simulink model "F16_dynamic_model_2019a"  (R2024b)
settings: Solver=ode3  StartTime=0.0  StopTime=1  FixedStep=1/1000  RelTol=1e-3
values from neighbouring files (symbols this model uses):
  f16data =     [f16aerodata.mat]
  f16engine =     [f16engine.mat]
undefined symbols (not defined in the file or in its folder): e0_0, e1_0, e2_0, e3_0, Earth, ft, m, s, WGS84
libraries: simulink_extras x11, simulink x7, aerosimlib x5, vrlib x3, sharedtransform x3, aerolibfltsims x3, slpidlib x3, aerolibconvert2 x2, aerolibutil x1, sharedutil x1, shared6dof x1, aerolibtransform2 x1
(part 2 of 3)

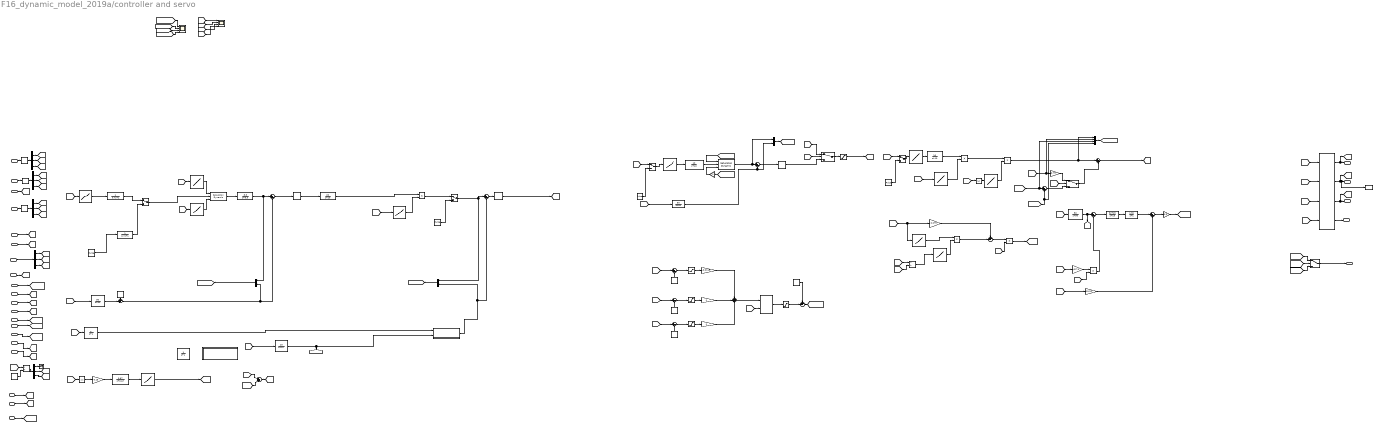
== system F16_dynamic_model_2019a/controller and servo  ==
  note: G limiters CAT 1
  note: Gain Scheduled Pitch Rate
  note: Scope
  note: Pitch Rate feedback
  note: Normal Acceleration feedback
  note: Adverse Yaw Prevent
  note: Stability Augmentation System
  note: INPUTS
  note: - PITCH CONTROL -
  note: POWER CONTROL
  note: SERVO (SIMPLE ACTUATORS)
  note: - RUDDER CONTROL -
  note: - ROLL CONTROL -
  note: Fake Alpha For High Roll to Alpha Limiter
  note: Roll Departure Preventation
  note: Aileron Rudder Interconnect ( ARI)
  note: NOT: Hız (160-255m/s arası) arttıkça
      |  command gain azalıyor.
  wbdots : Inport
  phithetapsi : Inport  Port=2
  h : Inport  Port=3
  wb (rad/s) : Inport  Port=4
  "Beta " : Inport  Port=5
  Vr : Inport  Port=6
  Ve : Inport  Port=7
  AoA : Inport  Port=8
  q_ah_des : Inport  Port=9
  dpower_ah : Inport  Port=10
  de_j : Inport  Port=11
  da_j : Inport  Port=12
  dr_j : Inport  Port=13
  dpower_j : Inport  Port=14
  "ah_check " : Inport  Port=15
  speedb : Inport  Port=16
  Ab(m/s2) : Inport  Port=17
  q_dyn : Inport  Port=18
  p_static : Inport  Port=19
  "turn_check " : Inport  Port=20
  1-D Lookup Table : Lookup_n-D  NumberOfTableDimensions=1  BreakpointsForDimension1=[-1, -0.2, 0.2, 1]  Table=[-30, 0, 0, 30]  ExtrapMethod=Clip  UseLastTableValue=on  InternalRulePriority=Speed  RndMeth=Simplest
  1-D Lookup Table1 : Lookup_n-D  NumberOfTableDimensions=1  BreakpointsForDimension1=[20, 30]  Table=[1, 0]  ExtrapMethod=Clip  UseLastTableValue=on  InternalRulePriority=Speed  RndMeth=Simplest
  1-D Lookup Table2 : Lookup_n-D  NumberOfTableDimensions=1  BreakpointsForDimension1=[3, 8.4]  Table=[0, 5.4]  ExtrapMethod=Clip  UseLastTableValue=on  InternalRulePriority=Speed  RndMeth=Simplest
  1-D Lookup Table3 : Lookup_n-D  NumberOfTableDimensions=1  BreakpointsForDimension1=[-10, 0, 10]  Table=[0, 1, 0]  ExtrapMethod=Clip  UseLastTableValue=on  InternalRulePriority=Speed  RndMeth=Simplest
  1-D Lookup Table4 : Lookup_n-D  NumberOfTableDimensions=1  BreakpointsForDimension1=[0.187, 1.129]  Table=[0, 1]  ExtrapMethod=Clip  UseLastTableValue=on  InternalRulePriority=Speed  RndMeth=Simplest
  Abs : Abs  SaturateOnIntegerOverflow=off
  Abs1 : Abs  SaturateOnIntegerOverflow=off
  Constant : Constant  Value=9.81
  Constant2 : Constant  Value=10500
  Constant3 : Constant  Value=15
  Constant4 : Constant  Value=5
  Constant5 : Constant  Value=308
  Control Signals : Scope  NumInputPorts=4
  Demux{,1..4} (5 alike) : Demux  Outputs=3
  Gain Scheduling Pitch Rate Feedback : Subsystem
  Gain1 : Gain  Gain=0.15
  Gain2 : Gain  Gain=-1
  Gain3 : Gain  Gain=0.75
  Manual Switch{,1..3} (4 alike) : ManualSwitch
  Multiply : Gain  Gain=-0.0115
  Multiply2 : Gain  Gain=0.075
  Multiply3 : Gain  Gain=4
  Multiply4 : Gain  Gain=4
  Multiply5 : Gain  Gain=1/57.3
  Multiply6 : Gain  Gain=19.32
  Multiply7 : Gain  Gain=0.5
  Mux : Mux  Inputs=2
  Mux1 : Mux  Inputs=2
  Mux2 : Mux  Inputs=2
  Mux3 : Mux
  PID Controller1 : slpidlib/PID Controller  Controller=PID  Form=Parallel  TimeDomain=Continuous-time  UseExternalTs=off  SampleTime=-1  IntegratorMethod=Forward Euler  FilterMethod=Forward Euler  ControllerParametersSource=internal  P=0.35  I=0.8  UseKiTs=off  D=0.04  UseExternalDerivativeSource=off  N=100  UseFilter=on  TunerSelectOption=Transfer Function Based (PID Tuner App)  InitialConditionSource=internal  InitialConditionForIntegrator=0  InitialConditionForFilter=0  DifferentiatorICPrevScaledInput=0  ExternalReset=none  TrackingMode=off  Kt=1  LimitOutput=on  SatLimitsSource=internal  UpperSaturationLimit=21.5  LowerSaturationLimit=-21.5  LinearizeAsGain=on  AntiWindupMode=clamping  Kb=1  LimitIntegrator=off  UpperIntegratorSaturationLimit=inf  LowerIntegratorSaturationLimit=-inf  POutMin=[]  POutMax=[]  IOutMin=[]  IOutMax=[]  DOutMin=[]  DOutMax=[]  NOutMin=[]  NOutMax=[]  SumOutMin=[]  SumOutMax=[]  SaturationOutMin=[]  SaturationOutMax=[]  PParamMin=[]  PParamMax=[]  IParamMin=[]  IParamMax=[]  DParamMin=[]  DParamMax=[]  NParamMin=[]  NParamMax=[]  KbParamMin=[]  KbParamMax=[]  KtParamMin=[]  KtParamMax=[]  KbOutMin=[]  KbOutMax=[]  KtOutMin=[]  KtOutMax=[]  IntegratorOutMin=[]  IntegratorOutMax=[]  FilterOutMin=[]  FilterOutMax=[]  SumI1OutMin=[]  SumI1OutMax=[]  SumI2OutMin=[]  SumI2OutMax=[]  SumI3OutMin=[]  SumI3OutMax=[]  SumI4OutMin=[]  SumI4OutMax=[]  SumDOutMin=[]  SumDOutMax=[]  DifferentiatorOutMin=[]  DifferentiatorOutMax=[]  FilterDiffOutCoefMin=[]  FilterDiffOutCoefMax=[]  ReciprocalOutMin=[]  ReciprocalOutMax=[]  SumDenOutMin=[]  SumDenOutMax=[]  SumNumOutMin=[]  SumNumOutMax=[]  DivideOutMin=[]  DivideOutMax=[]  UdiffTsProdOutMin=[]  UdiffTsProdOutMax=[]  NTsProdOutMin=[]  NTsProdOutMax=[]  UintegralTsProdOutMin=[]  UintegralTsProdOutMax=[]  UngainTsProdOutMin=[]  UngainTsProdOutMax=[]  ClampingZeroOutDataTypeStr=Inherit: Inherit via back propagation  ClampingZeroOutMin=[]  ClampingZeroOutMax=[]  FilterDenConstantOutDataTypeStr=Inherit: Inherit via back propagation  FilterDenConstantOutMin=[]  FilterDenConstantOutMax=[]  PCopyOutDataTypeStr=Inherit: Inherit via back propagation  PCopyOutMin=[]  PCopyOutMax=[]  NCopyOutDataTypeStr=Inherit: Inherit via back propagation  NCopyOutMin=[]  NCopyOutMax=[]  IntegratorContinuousStateAttributes=''  IntegratorStateMustResolveToSignalObject=off  IntegratorRTWStateStorageClass=Auto  FilterContinuousStateAttributes=''  FilterStateMustResolveToSignalObject=off  FilterRTWStateStorageClass=Auto  ParallelPVariant=InternalParameters  IdealPVariant=Disabled  IVariant=InternalParameters  DVariant=InternalParameters  IntegratorVariant=Continuous  SatVariant=Enabled  AWVariant=ContClampingParallel  PCopyVariant=Disabled  TRVariant=Disabled  FdbkBlocksVariant=Forward  IdealPFdbkVariant=Disabled  SatFdbkVariant=Disabled  DerivativeFilterVariant=ContFilter  NVariant=InternalParameters  NCopyVariant=Disabled  FilterICVariant=InternalICsFilter  IntegratorICVariant=InternalICs  ExternalResetVariant=Disabled  TRSumVariant=Passthrough  SumFdbkVariant=Disabled  SumVariant=Sum_PID  TsampFilterVariant=InternalTs  TsampNgainVariant=Passthrough  TsampIntegralVariant=Disabled_SignalSpec  ExternalSaturationOutDataTypeStr=Inherit: Same as second input  DerivativeSourceVariant=ErrorSignal  PreIntVariant=InternalPreInt
  PID de_cmd  5 step 2 : slpidlib/PID Controller  Controller=PID  Form=Parallel  TimeDomain=Continuous-time  UseExternalTs=off  SampleTime=-1  IntegratorMethod=Forward Euler  FilterMethod=Forward Euler  ControllerParametersSource=internal  P=2.5  I=5  UseKiTs=off  D=0.05  UseExternalDerivativeSource=off  N=100  UseFilter=on  TunerSelectOption=Transfer Function Based (PID Tuner App)  InitialConditionSource=internal  InitialConditionForIntegrator=0  InitialConditionForFilter=0  DifferentiatorICPrevScaledInput=0  ExternalReset=none  TrackingMode=off  Kt=1  LimitOutput=on  SatLimitsSource=internal  UpperSaturationLimit=25  LowerSaturationLimit=-25  LinearizeAsGain=on  AntiWindupMode=clamping  Kb=1  LimitIntegrator=off  UpperIntegratorSaturationLimit=inf  LowerIntegratorSaturationLimit=-inf  POutMin=[]  POutMax=[]  IOutMin=[]  IOutMax=[]  DOutMin=[]  DOutMax=[]  NOutMin=[]  NOutMax=[]  SumOutMin=[]  SumOutMax=[]  SaturationOutMin=[]  SaturationOutMax=[]  PParamMin=[]  PParamMax=[]  IParamMin=[]  IParamMax=[]  DParamMin=[]  DParamMax=[]  NParamMin=[]  NParamMax=[]  KbParamMin=[]  KbParamMax=[]  KtParamMin=[]  KtParamMax=[]  KbOutMin=[]  KbOutMax=[]  KtOutMin=[]  KtOutMax=[]  IntegratorOutMin=[]  IntegratorOutMax=[]  FilterOutMin=[]  FilterOutMax=[]  SumI1OutMin=[]  SumI1OutMax=[]  SumI2OutMin=[]  SumI2OutMax=[]  SumI3OutMin=[]  SumI3OutMax=[]  SumI4OutMin=[]  SumI4OutMax=[]  SumDOutMin=[]  SumDOutMax=[]  DifferentiatorOutMin=[]  DifferentiatorOutMax=[]  FilterDiffOutCoefMin=[]  FilterDiffOutCoefMax=[]  ReciprocalOutMin=[]  ReciprocalOutMax=[]  SumDenOutMin=[]  SumDenOutMax=[]  SumNumOutMin=[]  SumNumOutMax=[]  DivideOutMin=[]  DivideOutMax=[]  UdiffTsProdOutMin=[]  UdiffTsProdOutMax=[]  NTsProdOutMin=[]  NTsProdOutMax=[]  UintegralTsProdOutMin=[]  UintegralTsProdOutMax=[]  UngainTsProdOutMin=[]  UngainTsProdOutMax=[]  ClampingZeroOutDataTypeStr=Inherit: Inherit via back propagation  ClampingZeroOutMin=[]  ClampingZeroOutMax=[]  FilterDenConstantOutDataTypeStr=Inherit: Inherit via back propagation  FilterDenConstantOutMin=[]  FilterDenConstantOutMax=[]  PCopyOutDataTypeStr=Inherit: Inherit via back propagation  PCopyOutMin=[]  PCopyOutMax=[]  NCopyOutDataTypeStr=Inherit: Inherit via back propagation  NCopyOutMin=[]  NCopyOutMax=[]  IntegratorContinuousStateAttributes=''  IntegratorStateMustResolveToSignalObject=off  IntegratorRTWStateStorageClass=Auto  FilterContinuousStateAttributes=''  FilterStateMustResolveToSignalObject=off  FilterRTWStateStorageClass=Auto  ParallelPVariant=InternalParameters  IdealPVariant=Disabled  IVariant=InternalParameters  DVariant=InternalParameters  IntegratorVariant=Continuous  SatVariant=Enabled  AWVariant=ContClampingParallel  PCopyVariant=Disabled  TRVariant=Disabled  FdbkBlocksVariant=Forward  IdealPFdbkVariant=Disabled  SatFdbkVariant=Disabled  DerivativeFilterVariant=ContFilter  NVariant=InternalParameters  NCopyVariant=Disabled  FilterICVariant=InternalICsFilter  IntegratorICVariant=InternalICs  ExternalResetVariant=Disabled  TRSumVariant=Passthrough  SumFdbkVariant=Disabled  SumVariant=Sum_PID  TsampFilterVariant=InternalTs  TsampNgainVariant=Passthrough  TsampIntegralVariant=Disabled_SignalSpec  ExternalSaturationOutDataTypeStr=Inherit: Same as second input  DerivativeSourceVariant=ErrorSignal  PreIntVariant=InternalPreInt
  PID g cmd 1 : slpidlib/PID Controller  Controller=PID  Form=Parallel  TimeDomain=Continuous-time  UseExternalTs=off  SampleTime=-1  IntegratorMethod=Forward Euler  FilterMethod=Forward Euler  ControllerParametersSource=internal  P=5  I=2  UseKiTs=off  D=0  UseExternalDerivativeSource=off  N=100  UseFilter=on  TunerSelectOption=Transfer Function Based (PID Tuner App)  InitialConditionSource=internal  InitialConditionForIntegrator=0  InitialConditionForFilter=0  DifferentiatorICPrevScaledInput=0  ExternalReset=none  TrackingMode=off  Kt=1  LimitOutput=off  SatLimitsSource=internal  UpperSaturationLimit=inf  LowerSaturationLimit=-inf  LinearizeAsGain=on  AntiWindupMode=clamping  Kb=1  LimitIntegrator=off  UpperIntegratorSaturationLimit=inf  LowerIntegratorSaturationLimit=-inf  POutMin=[]  POutMax=[]  IOutMin=[]  IOutMax=[]  DOutMin=[]  DOutMax=[]  NOutMin=[]  NOutMax=[]  SumOutMin=[]  SumOutMax=[]  SaturationOutMin=[]  SaturationOutMax=[]  PParamMin=[]  PParamMax=[]  IParamMin=[]  IParamMax=[]  DParamMin=[]  DParamMax=[]  NParamMin=[]  NParamMax=[]  KbParamMin=[]  KbParamMax=[]  KtParamMin=[]  KtParamMax=[]  KbOutMin=[]  KbOutMax=[]  KtOutMin=[]  KtOutMax=[]  IntegratorOutMin=[]  IntegratorOutMax=[]  FilterOutMin=[]  FilterOutMax=[]  SumI1OutMin=[]  SumI1OutMax=[]  SumI2OutMin=[]  SumI2OutMax=[]  SumI3OutMin=[]  SumI3OutMax=[]  SumI4OutMin=[]  SumI4OutMax=[]  SumDOutMin=[]  SumDOutMax=[]  DifferentiatorOutMin=[]  DifferentiatorOutMax=[]  FilterDiffOutCoefMin=[]  FilterDiffOutCoefMax=[]  ReciprocalOutMin=[]  ReciprocalOutMax=[]  SumDenOutMin=[]  SumDenOutMax=[]  SumNumOutMin=[]  SumNumOutMax=[]  DivideOutMin=[]  DivideOutMax=[]  UdiffTsProdOutMin=[]  UdiffTsProdOutMax=[]  NTsProdOutMin=[]  NTsProdOutMax=[]  UintegralTsProdOutMin=[]  UintegralTsProdOutMax=[]  UngainTsProdOutMin=[]  UngainTsProdOutMax=[]  ClampingZeroOutDataTypeStr=Inherit: Inherit via back propagation  ClampingZeroOutMin=[]  ClampingZeroOutMax=[]  FilterDenConstantOutDataTypeStr=Inherit: Inherit via back propagation  FilterDenConstantOutMin=[]  FilterDenConstantOutMax=[]  PCopyOutDataTypeStr=Inherit: Inherit via back propagation  PCopyOutMin=[]  PCopyOutMax=[]  NCopyOutDataTypeStr=Inherit: Inherit via back propagation  NCopyOutMin=[]  NCopyOutMax=[]  IntegratorContinuousStateAttributes=''  IntegratorStateMustResolveToSignalObject=off  IntegratorRTWStateStorageClass=Auto  FilterContinuousStateAttributes=''  FilterStateMustResolveToSignalObject=off  FilterRTWStateStorageClass=Auto  ParallelPVariant=InternalParameters  IdealPVariant=Disabled  IVariant=InternalParameters  DVariant=InternalParameters  IntegratorVariant=Continuous  SatVariant=Disabled  AWVariant=Passthrough  PCopyVariant=Disabled  TRVariant=Disabled  FdbkBlocksVariant=Forward  IdealPFdbkVariant=Disabled  SatFdbkVariant=Disabled  DerivativeFilterVariant=ContFilter  NVariant=InternalParameters  NCopyVariant=Disabled  FilterICVariant=InternalICsFilter  IntegratorICVariant=InternalICs  ExternalResetVariant=Disabled  TRSumVariant=Passthrough  SumFdbkVariant=Disabled  SumVariant=Sum_PID  TsampFilterVariant=InternalTs  TsampNgainVariant=Passthrough  TsampIntegralVariant=Disabled_SignalSpec  ExternalSaturationOutDataTypeStr=Inherit: Same as second input  DerivativeSourceVariant=ErrorSignal  PreIntVariant=InternalPreInt
  Product{,1,4,6..8} (6 alike) : Product
  Product2 : Product  Inputs=*/
  Product5 : Product  Inputs=*/
  Pulse Generator : DiscretePulseGenerator  PulseType=Time based  Period=100  PulseWidth=2.5  PhaseDelay=3
  Pulse Generator1 : DiscretePulseGenerator  PulseType=Time based  Period=100  PulseWidth=2.5  PhaseDelay=3
  Pulse Generator2 : DiscretePulseGenerator  PulseType=Time based  Amplitude=2  Period=100  PulseWidth=2  PhaseDelay=3
  Pulse Generator3 : DiscretePulseGenerator  PulseType=Time based  Amplitude=3  Period=100  PulseWidth=2  PhaseDelay=3
  Radians to Degrees : simulink_extras/Transformations/Radians to Degrees
  Radians to Degrees1 : simulink_extras/Transformations/Radians to Degrees
  Radians to Degrees2 : simulink_extras/Transformations/Radians to Degrees
  Saturation Dynamic : simulink/Discontinuities/Saturation Dynamic  OutMin=[]  OutMax=[]  OutDataTypeStr=Inherit: Same as second input  OutDataType=fixdt(1, 16)  OutScaling=2^-10  DoSatur=off
  Saturation Dynamic1 : simulink/Discontinuities/Saturation Dynamic  OutMin=[]  OutMax=[]  OutDataTypeStr=Inherit: Same as second input  OutDataType=fixdt(1, 16)  OutScaling=2^-10  DoSatur=off
  Saturation1 : Saturate  UpperLimit=21.5  LowerLimit=-21.5
  Saturation3 : Saturate  UpperLimit=0  LowerLimit=-inf
  Saturation4 : Saturate  UpperLimit=inf  LowerLimit=0
  Saturation5 : Saturate  UpperLimit=inf  LowerLimit=0
  Saturation6 : Saturate  UpperLimit=228  LowerLimit=0
  State Signals : Scope  NumInputPorts=4
  Subsystem2 : Subsystem
  Sum : Sum  Inputs=|++
  Sum1 : Sum  Inputs=|++|
  Sum{2,4,6,8,10..11,13} (7 alike) : Sum  Inputs=|+-
  Sum12 : Sum  Inputs=+-|
  Sum14 : Sum  Inputs=|++
  Sum15 : Sum  Inputs=|++
  Sum16 : Sum  Inputs=++|
  Sum7 : Sum  Inputs=+-|
  Sum9 : Sum  Inputs=+++
  Switch : Switch  Criteria=u2 > Threshold  SaturateOnIntegerOverflow=off  InputSameDT=off
  Switch2 : Switch  Threshold=30  SaturateOnIntegerOverflow=off  InputSameDT=off
  Switch3 : Switch  Threshold=29  SaturateOnIntegerOverflow=off  InputSameDT=off
  Terminator : Terminator
  To Workspace : ToWorkspace  VariableName=de_act  SampleTime=-1
  Transfer Fcn1 : TransferFcn  Numerator=[10]  Denominator=[1 10]
  Transfer Fcn10 : TransferFcn  Numerator=[10]  Denominator=[1 10]
  Transfer Fcn12 : TransferFcn  Numerator=[50]  Denominator=[1 50]
  Transfer Fcn13 : TransferFcn  Denominator=[0.7 1]
  Transfer Fcn16 : TransferFcn  Numerator=[20]  Denominator=[1 20]
  Transfer Fcn17 : TransferFcn  Numerator=[8.3]  Denominator=[1 8.3]
  Transfer Fcn18 : TransferFcn  Numerator=[1 ]  Denominator=[1 1]
  Transfer Fcn2 : TransferFcn  Numerator=[3 15]  Denominator=[1 15]
  Transfer Fcn20 : TransferFcn  Numerator=[50]  Denominator=[1 50]
  Transfer Fcn3 : TransferFcn  Numerator=[10]  Denominator=[1 10]
  Transfer Fcn4 : TransferFcn  Denominator=[0.7 1]
  Transfer Fcn5 : TransferFcn  Numerator=[0.67]  Denominator=[1 0.67]
  Transfer Fcn6 : TransferFcn  Numerator=[1 0]  Denominator=[1 1]
  Transfer Fcn7 : TransferFcn  Numerator=[50]  Denominator=[1 50]
  Transfer Fcn8 : TransferFcn  Numerator=[1.5 0]  Denominator=[1 1]
  "allowable g " : Lookup_n-D  NumberOfTableDimensions=1  BreakpointsForDimension1=[15, 20, 25]  Table=[8, 6.3, 0]  ExtrapMethod=Clip  UseLastTableValue=on  InternalRulePriority=Speed  RndMeth=Simplest
  "bias g " : Constant  Value=0
  "negative g limit (q N/m, g)" : Lookup_n-D  NumberOfTableDimensions=1  BreakpointsForDimension1=[2000, 9000]  Table=[-1, -4]  ExtrapMethod=Clip  UseLastTableValue=on  InternalRulePriority=Speed  RndMeth=Simplest
  pitch command gradient (g) : Lookup_n-D  NumberOfTableDimensions=1  BreakpointsForDimension1=[-1, -0.375, -0.125, 0.05, 0.2, 1]  Table=[-4, -0.6, 0, 0, 0.5, 10]  ExtrapMethod=Clip  UseLastTableValue=on  InternalRulePriority=Speed  RndMeth=Simplest
  pitch-loop gain (q N/m) : Lookup_n-D  NumberOfTableDimensions=1  BreakpointsForDimension1=[16000, 42000]  Table=[1, 0.4]  ExtrapMethod=Clip  UseLastTableValue=on  InternalRulePriority=Speed  RndMeth=Simplest
  roll command gradient (deg/sec) : Lookup_n-D  NumberOfTableDimensions=1  BreakpointsForDimension1=[-1, -0.625, -0.3125, -0.1, 0.1, 0.3125, 0.625, 1]  Table=[-300, -90, -40, 0, 0, 40, 90, 300]  ExtrapMethod=Clip  UseLastTableValue=on  InternalRulePriority=Speed  RndMeth=Simplest
  roll rate limiter (deg/s) : Lookup_n-D  NumberOfTableDimensions=1  BreakpointsForDimension1=[20, 40]  Table=[1, 0]  ExtrapMethod=Clip  UseLastTableValue=on  InternalRulePriority=Speed  RndMeth=Simplest
  scheduled gain : Subsystem
  "servo " : Subsystem
  da_act : Outport
  de_act : Outport  Port=2
  dr_act : Outport  Port=3
  dpower : Outport  Port=4
  dsb_act : Outport  Port=5
  wires:
  Demux/2 -> [theta]
  Demux/1 -> [phi]
  Demux/3 -> [psi]
  phithetapsi/1 -> Radians to Degrees/1
  wb (rad/s)/1 -> Radians to Degrees2/1
  Demux1/3 -> [r]
  Demux1/1 -> [p]
  Demux1/2 -> [q]
  h/1 -> [altitude]
  Demux2/2 -> [Vy]
  Ve/1 -> Demux2/1
  Demux2/1 -> [Vx]
  Demux2/3 -> [Vz]
  "Beta "/1 -> [beta]
  Vr/1 -> [Vr]
  AoA/1 -> [AoA]
  dr_j/1 -> [dr_j]
  da_j/1 -> [da_j]
  de_j/1 -> [de_j]
  q_ah_des/1 -> [q_ah_desired]
  "servo "/3(Out3) -> [dr_act], dr_act/1
  "servo "/1(Out1) -> [da_act], da_act/1
  [da_c] -> "servo "/1(In1)
  [dr_c] -> "servo "/3(In3)
  dpower_ah/1 -> [dpower_ah]
  dpower_j/1 -> [dpower_j]
  [ah_check] -> Switch/2
  [dpower_ah] -> Switch/1
  [dpower_j] -> Switch/3
  Switch/1 -> dpower/1
  "ah_check "/1 -> [ah_check]
  Radians to Degrees/1 -> Demux/1
  Demux3/2 -> [thetado]
  Demux3/3 -> [psidot]
  Demux3/1 -> [phidot]
  Radians to Degrees1/1 -> Demux3/1
  wbdots/1 -> Radians to Degrees1/1
  PID Controller1/1 -> Switch2/3
  [p] -> Transfer Fcn20/1  "feedback"
  roll command gradient (deg/sec)/1 -> Transfer Fcn1/1
  [AoA] -> 1-D Lookup Table1/1
  Product/1 -> Product1/1
  roll rate limiter (deg/s)/1 -> Product1/2
  [p] -> Abs/1
  1-D Lookup Table1/1 -> Product/2
  Abs/1 -> roll rate limiter (deg/s)/1
  1-D Lookup Table/1 -> Transfer Fcn3/1
  Radians to Degrees2/1 -> Demux1/1
  [dr_j] -> Manual Switch1/1
  speedb/1 -> [dsb_j]
  [dsb_j] -> "servo "/4(In4)
  "servo "/4(Output) -> dsb_act/1
  Ab(m/s2)/1 -> [Ab]
  Constant/1 -> Product2/2
  [Ab] -> Product2/1
  Product2/1 -> Demux4/1
  Demux4/3 -> [a_n]
  Demux4/1 -> Terminator/1
  Demux4/2 -> [a_y]
  q_dyn/1 -> [q_dyn]
  [AoA] -> Sum1/1
  [dAoA_p] -> Sum1/2
  Sum1/1 -> [AoA_t]
  Abs1/1 -> Gain1/1
  Gain1/1 -> Transfer Fcn5/1
  Transfer Fcn5/1 -> 1-D Lookup Table2/1
  1-D Lookup Table2/1 -> [dAoA_p]
  [p] -> Abs1/1
  [q] -> Transfer Fcn6/1
  [de_act] -> Sum11/1
  Sum8/1 -> Saturation3/1
  Sum9/1 -> scheduled gain/1(In1)
  [AoA] -> Sum10/1
  Constant3/1 -> Sum10/2
  Constant4/1 -> Sum11/2
  Sum12/1 -> [p_com_max]
  Sum11/1 -> Saturation5/1
  Multiply3/1 -> Sum9/2
  Saturation6/1 -> Sum12/2
  [q_dyn] -> Sum8/1
  Multiply4/1 -> Sum9/3
  Sum10/1 -> Saturation4/1
  Constant2/1 -> Sum8/2
  Saturation5/1 -> Multiply4/1
  [p] -> scheduled gain/2(In2)
  Saturation4/1 -> Multiply3/1
  Constant5/1 -> Sum12/1
  scheduled gain/1(Out1) -> Saturation6/1
  Multiply/1 -> Sum9/1
  Saturation3/1 -> Multiply/1
  [p_com_max] -> Saturation Dynamic1/1
  [p_com_max] -> Gain2/1
  Gain2/1 -> Saturation Dynamic1/3
  Saturation Dynamic1/1 -> Mux/1, Sum2/1  "Roll Rate Cmd"
  [AoA] -> Switch2/2
  Switch2/1 -> Saturation1/1
  [r_f] -> Switch2/1
  Saturation1/1 -> [da_c]
  [AoA] -> Switch3/2
  Product1/1 -> Mux3/1, Sum/1  "Rudder Angle Cmd"
  Gain3/1 -> Switch3/1
  [q_dyn] -> Product5/1
  Product5/1 -> 1-D Lookup Table4/1
  1-D Lookup Table4/1 -> Product4/2
  Multiply2/1 -> Sum7/1
  1-D Lookup Table3/1 -> Product4/1
  [da_act] -> Product6/2
  Sum7/1 -> Product6/1
  Product4/1 -> Sum7/2
  Product6/1 -> [yaw_ari]
  [AoA_t] -> Multiply2/1, 1-D Lookup Table3/1
  p_static/1 -> [p_s]
  [p_s] -> Product5/2
  Transfer Fcn7/1 -> Sum13/1, [r_f]
  [r] -> Transfer Fcn7/1
  Product7/1 -> Sum13/2
  [p] -> Multiply5/1
  Multiply5/1 -> Product7/1
  [AoA_t] -> Product7/2
  [a_y] -> Multiply6/1
  Sum13/1 -> Transfer Fcn2/1
  Transfer Fcn2/1 -> Transfer Fcn8/1
  Transfer Fcn8/1 -> Sum14/1
  Multiply6/1 -> Sum14/2
  Sum14/1 -> Multiply7/1
  Multiply7/1 -> [yaw_sas]
  [yaw_ari] -> Mux3/3, Sum15/1  "ARI Feedback"
  [yaw_sas] -> Mux3/4, Sum15/2  "SAS Feedback"
  Sum15/1 -> Switch3/3
  [r_f] -> Mux3/2, Gain3/1  "Rudder Angle"
  [de_c] -> "servo "/2(In2)
  [de_j] -> pitch command gradient (g)/1
  "turn_check "/1 -> [turn_check]
  Mux/1 -> [rollratesignal]
  Mux1/1 -> [pitchratesignal]
  Mux2/1 -> [G_cmds]
  Switch3/1 -> Sum/2  "Rudder Angle"
  Mux3/1 -> [yawdegsignal]
  [G_cmds] -> Control Signals/1
  [rollratesignal] -> Control Signals/3
  [yawdegsignal] -> Control Signals/4
  [AoA] -> State Signals/1
  [beta] -> State Signals/2
  [Vr] -> State Signals/3
  [altitude] -> State Signals/4
  Sum2/1 -> PID Controller1/1
  Transfer Fcn3/1 -> Product/1
  Sum16/1 -> Sum4/2, Mux2/2  "Normal acc feedback"
  [pitchratesignal] -> Control Signals/2
  Sum/1 -> [dr_c]
  "bias g "/1 -> Sum16/1
  [AoA_t] -> Transfer Fcn10/1  "feedback"
  Transfer Fcn10/1 -> Subsystem2/2(aoa), [aoasignal]  "feedback"
  Transfer Fcn20/1 -> Sum2/2, Mux/2  "Roll Rate Feedback"
  Transfer Fcn1/1 -> Saturation Dynamic1/2
  Manual Switch2/1 -> Mux1/1, Sum6/1  "Pitch Rate Cmd"
  pitch-loop gain (q N/m)/1 -> Product8/2
  Transfer Fcn16/1 -> Product8/1
  [q_dyn] -> pitch-loop gain (q N/m)/1
  [AoA_t] -> "allowable g "/1
  Transfer Fcn17/1 -> Mux2/1, Sum4/1  "G command"
  Transfer Fcn4/1 -> Manual Switch3/1
  "allowable g "/1 -> Saturation Dynamic/1
  "negative g limit (q N/m, g)"/1 -> Saturation Dynamic/3
  [q_dyn] -> "negative g limit (q N/m, g)"/1
  [a_n] -> Transfer Fcn12/1  "feedback"
  "servo "/2(Out2) -> [de_act], To Workspace/1, de_act/1
  Transfer Fcn12/1 -> Sum16/2  "feedback"
  Sum4/1 -> PID g cmd 1/1
  Subsystem2/1(Out1) -> Sum6/2, Mux1/2  "Pitch rate feedback"
  Transfer Fcn6/1 -> Subsystem2/1(Pitch rate feedback)  "Pitch rate feedback"
  Saturation Dynamic/1 -> Transfer Fcn17/1  "G command"
  Transfer Fcn13/1 -> Manual Switch3/2
  Pulse Generator3/1 -> Transfer Fcn13/1  "test step"
  Pulse Generator2/1 -> Manual Switch2/2
  Product8/1 -> Manual Switch2/1
  PID g cmd 1/1 -> Transfer Fcn16/1
  Manual Switch3/1 -> Saturation Dynamic/2
  PID de_cmd  5 step 2/1 -> [de_c]
  Sum6/1 -> PID de_cmd  5 step 2/1
  [da_j] -> Manual Switch/1
  Manual Switch/1 -> roll command gradient (deg/sec)/1
  Pulse Generator/1 -> Manual Switch/2
  Manual Switch1/1 -> 1-D Lookup Table/1
  Pulse Generator1/1 -> Manual Switch1/2
  pitch command gradient (g)/1 -> Transfer Fcn4/1

== system F16_dynamic_model_2019a/MODEL/6-DOF Model Body Euler ==
  F_xyz (N) : Inport
  mass : Inport  Port=2
  M_xyz (Nm) : Inport  Port=3
  Angular_Accel : Subsystem
  Constant : Constant  Value=[180 0 0]  VectorParams1D=off
  Constant1 : Constant
  Inertia : Subsystem
  Integrator1 : Integrator
  Product : Product  Inputs=*/
  Subsystem : Subsystem
  Sum : Sum
  Transpose : Math  Operator=transpose  SignedPower=on
  V_body : Integrator  InitialConditionSource=external  InitialCondition=[10 20 0]
  body_axis_coriolis_accel : Subsystem
  "p q r " : Integrator  InitialCondition=[0 0 0]
  "transform to Inertial axes " : shared6dof/6DOF (Euler Angles)/transform to Inertial axes   SystemSampleTime=-1  Latency=0  AutoFrameSizeCalculation=off
      settings: SourceProductName=Aerospace Blockset
  Ve_flat (m/s) : Outport  Unit=m/s
  Xe_flat (m) : Outport  Port=2  Unit=m
  Euler Angles (rad) : Outport  Port=3  Unit=rad
  DCM : Outport  Port=4
  Vb (m/s) : Outport  Port=5  Unit=m/s
  p q r (rad/s) : Outport  Port=6  Unit=rad/s
  pdot qdot rdot (rad/s^2) : Outport  Port=7  Unit=rad/s^2
  Ab (m/s^2) : Outport  Port=8  Unit=m/s^2
  wires:
  F_xyz (N)/1 -> Product/1
  mass/1 -> Product/2
  Product/1 -> Sum/1
  body_axis_coriolis_accel/1(Accel_coriolis_body) -> Sum/2
  Sum/1 -> Ab (m/s^2)/1, V_body/1
  M_xyz (Nm)/1 -> Angular_Accel/1(Moments)
  "p q r "/1 -> p q r (rad/s)/1, body_axis_coriolis_accel/2(p q r), Angular_Accel/3(p q r), Subsystem/1(p q r)
  Angular_Accel/1("pdot qdot rdot ") -> pdot qdot rdot (rad/s^2)/1, "p q r "/1
  Subsystem/2(Euler) -> Euler Angles (rad)/1
  V_body/1 -> Vb (m/s)/1, body_axis_coriolis_accel/1(u v w), "transform to Inertial axes "/1
  "transform to Inertial axes "/1 -> Ve_flat (m/s)/1, Integrator1/1
  Integrator1/1 -> Xe_flat (m)/1
  Constant/1 -> V_body/2
  Constant1/1 -> Inertia/1(In1)
  Inertia/1(inertia matrix) -> Angular_Accel/2(Inertia)
  Transpose/1 -> "transform to Inertial axes "/2
  Subsystem/1(DCM1) -> DCM/1, Transpose/1

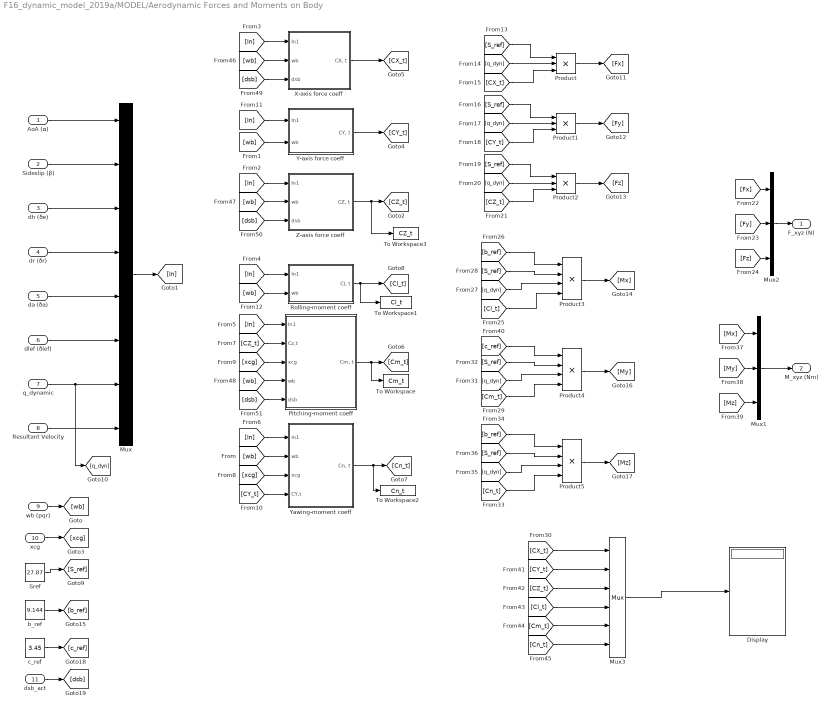
== system F16_dynamic_model_2019a/MODEL/Aerodynamic Forces and Moments on Body ==
  AoA (α) : Inport
  Sideslip (β) : Inport  Port=2
  dh (δe) : Inport  Port=3
  dr (δr) : Inport  Port=4
  da (δa) : Inport  Port=5
  dlef (δlef) : Inport  Port=6
  q_dynamic : Inport  Port=7
  Resultant Velocity : Inport  Port=8
  wb (pqr) : Inport  Port=9
  "xcg " : Inport  Port=10
  "dsb_act " : Inport  Port=11
  Display : Display
  Mux : Mux  Inputs=8
  Mux1 : Mux  Inputs=3
  Mux2 : Mux  Inputs=3
  Mux3 : Mux  Inputs=6
  Pitching-moment coeff : Subsystem
  Product : Product  Inputs=3
  Product1 : Product  Inputs=3
  Product2 : Product  Inputs=3
  Product3 : Product  Inputs=4
  Product4 : Product  Inputs=4
  Product5 : Product  Inputs=4
  Rolling-moment coeff : Subsystem
  Sref : Constant  Value=27.87
  To Workspace : ToWorkspace  VariableName=Cm_t  SampleTime=-1
  To Workspace1 : ToWorkspace  VariableName=Cl_t  SampleTime=-1
  To Workspace2 : ToWorkspace  VariableName=Cn_t  SampleTime=-1
  To Workspace3 : ToWorkspace  VariableName=CZ_t  SampleTime=-1
  X-axis force coeff : Subsystem
  Y-axis force coeff : Subsystem
  Yawing-moment coeff : Subsystem
  Z-axis force coeff : Subsystem
  b_ref : Constant  Value=9.144
  c_ref : Constant  Value=3.45
  F_xyz (N) : Outport
  M_xyz (Nm) : Outport  Port=2
  wires:
  AoA (α)/1 -> Mux/1
  Sideslip (β)/1 -> Mux/2
  dh (δe)/1 -> Mux/3
  dr (δr)/1 -> Mux/4
  da (δa)/1 -> Mux/5
  dlef (δlef)/1 -> Mux/6
  q_dynamic/1 -> [q_dyn], Mux/7
  Resultant Velocity/1 -> Mux/8
  wb (pqr)/1 -> [wb]
  [wb] -> Yawing-moment coeff/2(wb)
  [wb] -> Y-axis force coeff/2("wb ")
  Mux/1 -> [In]
  [In] -> Z-axis force coeff/1(In1)
  [In] -> X-axis force coeff/1(In1)
  [In] -> Yawing-moment coeff/1(In1)
  [In] -> Pitching-moment coeff/1(In1)
  Z-axis force coeff/1("CZ, t") -> To Workspace3/1, [CZ_t]
  [CZ_t] -> Pitching-moment coeff/2(Cz,t)
  "xcg "/1 -> [xcg]
  [xcg] -> Yawing-moment coeff/3(xcg)
  [xcg] -> Pitching-moment coeff/3(xcg)
  Y-axis force coeff/1("CY, t") -> [CY_t]
  X-axis force coeff/1("CX, t") -> [CX_t]
  Pitching-moment coeff/1("Cm, t") -> To Workspace/1, [Cm_t]
  Yawing-moment coeff/1("Cn, t") -> To Workspace2/1, [Cn_t]
  [CY_t] -> Yawing-moment coeff/4(CY,t)
  [In] -> Y-axis force coeff/1(In1)
  [In] -> Rolling-moment coeff/1(In1)
  Rolling-moment coeff/1("Cl, t") -> [Cl_t], To Workspace1/1
  [wb] -> Rolling-moment coeff/2(wb)
  Mux2/1 -> F_xyz (N)/1
  Sref/1 -> [S_ref]
  [S_ref] -> Product/1
  [q_dyn] -> Product/2
  [CX_t] -> Product/3
  Product/1 -> [Fx]
  Product1/1 -> [Fy]
  [q_dyn] -> Product1/2
  [CY_t] -> Product1/3
  [S_ref] -> Product1/1
  Product2/1 -> [Fz]
  [q_dyn] -> Product2/2
  [CZ_t] -> Product2/3
  [S_ref] -> Product2/1
  [Fx] -> Mux2/1
  [Fy] -> Mux2/2
  [Fz] -> Mux2/3
  Product3/1 -> [Mx]
  [Cl_t] -> Product3/4
  b_ref/1 -> [b_ref]
  [b_ref] -> Product3/1
  [S_ref] -> Product3/2
  [q_dyn] -> Product3/3
  [c_ref] -> Product4/1
  [S_ref] -> Product4/2
  [q_dyn] -> Product4/3
  Product4/1 -> [My]
  [b_ref] -> Product5/1
  [S_ref] -> Product5/2
  [q_dyn] -> Product5/3
  Product5/1 -> [Mz]
  [Cn_t] -> Product5/4
  [Cm_t] -> Product4/4
  [Mx] -> Mux1/1
  [My] -> Mux1/2
  [Mz] -> Mux1/3
  c_ref/1 -> [c_ref]
  [CX_t] -> Mux3/1
  [CY_t] -> Mux3/2
  [CZ_t] -> Mux3/3
  [Cl_t] -> Mux3/4
  [Cm_t] -> Mux3/5
  [Cn_t] -> Mux3/6
  Mux3/1 -> Display/1
  [wb] -> X-axis force coeff/2(wb)
  [wb] -> Z-axis force coeff/2(wb)
  [wb] -> Pitching-moment coeff/4(wb)
  "dsb_act "/1 -> [dsb]
  [dsb] -> X-axis force coeff/3(dsb)
  [dsb] -> Z-axis force coeff/3(dsb)
  [dsb] -> Pitching-moment coeff/5(dsb)
  Mux1/1 -> M_xyz (Nm)/1

== system F16_dynamic_model_2019a/MODEL/Air  ==
  Vb : Inport
  Xe_flat : Inport  Port=2
  Add4 : Sum  Inputs=+++
  Constant : Constant  Value=-5000
  Demux : Demux  Outputs=3
  Display : Display
  Display1 : Display
  Flat Earth to LLA : aerolibtransform2/Flat Earth to LLA  units=Metric (MKS)  ptype=Earth (WGS84)  F=1/298.257223563  R=6378137  LL0=[41.028407,28.898297]  psi=0
  Gain9 : Gain  Gain=0.5
  ISA Atmosphere Model : aerolibatmos2/ISA Atmosphere Model  custom=off  g=9.80665  gamma=1.4  R=287.0531  L=0.0065  h_trop=11000  h_strat=20000  rho0=1.225  P0=101325  T0=288.15  h0=0
      settings: SourceProductName=Aerospace Blockset
  Mux : Mux  Inputs=2
  Product6 : Product
  Sqrt : Sqrt
  Square{,1..3} (4 alike) : Math  Operator=square  SignedPower=on
  Terminator1 : Terminator
  Terminator2 : Terminator
  "q_dyn " : Outport
  Vr : Outport  Port=2
  mu I h : Outport  Port=3
  "altitude " : Outport  Port=4
  p_s : Outport  Port=5
  wires:
  Gain9/1 -> Product6/1
  Demux/3 -> Square2/1
  Flat Earth to LLA/2 -> ISA Atmosphere Model/1, "altitude "/1, Mux/2
  Product6/1 -> "q_dyn "/1
  Square2/1 -> Add4/3
  Square1/1 -> Add4/2
  Demux/1 -> Square/1
  Square/1 -> Add4/1
  Add4/1 -> Sqrt/1
  Demux/2 -> Square1/1
  [rho] -> Product6/2
  Constant/1 -> Flat Earth to LLA/2
  ISA Atmosphere Model/4 -> [rho]
  Square3/1 -> Gain9/1
  Sqrt/1 -> Display1/1, Vr/1, Square3/1
  Vb/1 -> Display/1, Demux/1
  Xe_flat/1 -> Flat Earth to LLA/1
  Flat Earth to LLA/1 -> Mux/1
  ISA Atmosphere Model/1 -> Terminator1/1
  ISA Atmosphere Model/2 -> Terminator2/1
  ISA Atmosphere Model/3 -> p_s/1
  Mux/1 -> mu I h/1

== system F16_dynamic_model_2019a/MODEL/Subsystem ==
  Vb : Inport
  Atan : Trigonometry  Operator=atan
  Atan1 : Trigonometry  Operator=atan
  Demux : Demux  Outputs=3
  Divide : Product  Inputs=*/
  Divide1 : Product  Inputs=*/
  Radians to Degrees : simulink_extras/Transformations/Radians to Degrees
  Radians to Degrees1 : simulink_extras/Transformations/Radians to Degrees
  AoA (deg) : Outport
  Sideslip (beta) (deg) : Outport  Port=2
  wires:
  Divide1/1 -> Atan1/1
  Radians to Degrees1/1 -> Sideslip (beta) (deg)/1
  Demux/2 -> Divide1/1
  Atan/1 -> Radians to Degrees/1
  Divide/1 -> Atan/1
  Vb/1 -> Demux/1
  Atan1/1 -> Radians to Degrees1/1
  Demux/3 -> Divide/1
  Demux/1 -> Divide1/2, Divide/2
  Radians to Degrees/1 -> AoA (deg)/1

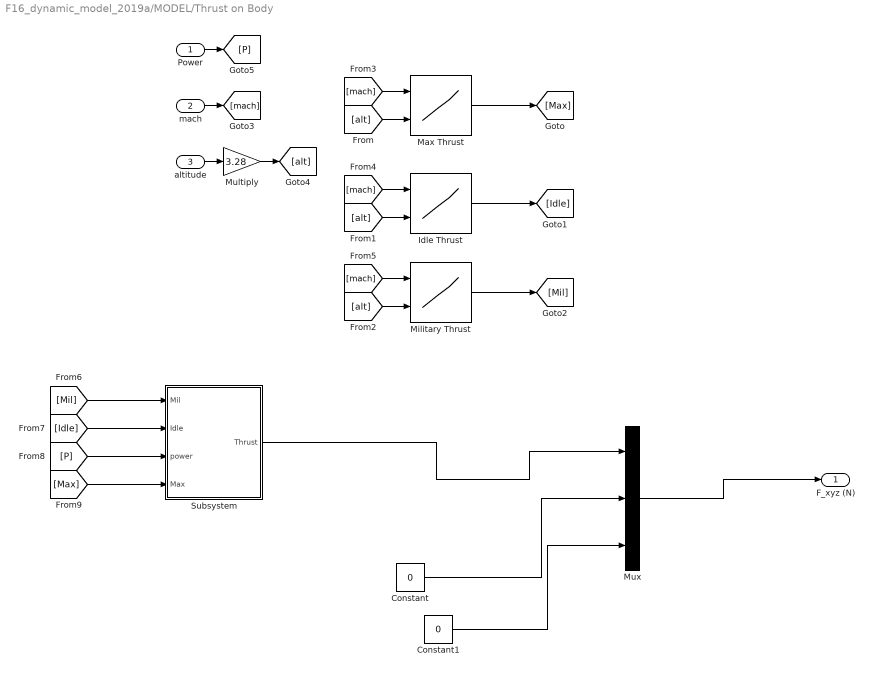
== system F16_dynamic_model_2019a/MODEL/Thrust on Body  ==
  Power : Inport
  mach : Inport  Port=2
  altitude : Inport  Port=3
  Constant : Constant  Value=0
  Constant1 : Constant  Value=0
  Idle Thrust : Lookup_n-D  BreakpointsForDimension1=f16engine.Ma  BreakpointsForDimension2=f16engine.alt  BreakpointsForDimension3=[5, 7]  Table=f16engine.Idle  ExtrapMethod=Clip  DiagnosticForOutOfRangeInput=Warning  InternalRulePriority=Speed  RndMeth=Simplest
      settings: InputPortMap=u0,u1
  Max Thrust : Lookup_n-D  BreakpointsForDimension1=f16engine.Ma  BreakpointsForDimension2=f16engine.alt  BreakpointsForDimension3=[5, 7]  Table=f16engine.Max  ExtrapMethod=Clip  DiagnosticForOutOfRangeInput=Warning  InternalRulePriority=Speed  RndMeth=Simplest
      settings: InputPortMap=u0,u1
  Military Thrust : Lookup_n-D  BreakpointsForDimension1=f16engine.Ma  BreakpointsForDimension2=f16engine.alt  BreakpointsForDimension3=[5, 7]  Table=f16engine.Mil  ExtrapMethod=Clip  DiagnosticForOutOfRangeInput=Warning  InternalRulePriority=Speed  RndMeth=Simplest
      settings: InputPortMap=u0,u1
  Multiply : Gain  Gain=3.28
  Mux : Mux  Inputs=3
  Subsystem : Subsystem
  F_xyz (N) : Outport
  wires:
  Idle Thrust/1 -> [Idle]
  Military Thrust/1 -> [Mil]
  mach/1 -> [mach]
  altitude/1 -> Multiply/1
  Power/1 -> [P]
  [Mil] -> Subsystem/1(Mil)
  [Idle] -> Subsystem/2(Idle)
  [P] -> Subsystem/3(power)
  [Max] -> Subsystem/4(Max)
  Mux/1 -> F_xyz (N)/1
  Subsystem/1(Thrust) -> Mux/1
  Constant/1 -> Mux/2
  Constant1/1 -> Mux/3
  Max Thrust/1 -> [Max]
  [mach] -> Military Thrust/1
  [alt] -> Military Thrust/2
  [mach] -> Idle Thrust/1
  [alt] -> Idle Thrust/2
  [alt] -> Max Thrust/2
  [mach] -> Max Thrust/1
  Multiply/1 -> [alt]

== system F16_dynamic_model_2019a/MODEL/dlef ==
  "p_s " : Inport
  AoA : Inport  Port=2
  "q_dyn " : Inport  Port=3
  Constant : Constant  Value=1.45
  Multiply : Gain  Gain=1.38
  Multiply1 : Gain  Gain=-9.05
  Product : Product  Inputs=*/
  Simple Actuator leading-edge flap (1st-order dynamics) : aerosimlib/Actuators/Simple Actuator (1st-order dynamics)  MaxRate=25  CountRange=[0 1024]  ActRange=[0 25]  Lag=0.136
  Sum : Sum  Inputs=+++
  Transfer Fcn : TransferFcn  Numerator=[2 7.25]  Denominator=[1 7.25]
  dlef : Outport
  wires:
  AoA/1 -> Transfer Fcn/1
  Transfer Fcn/1 -> Multiply/1
  "q_dyn "/1 -> Product/1
  "p_s "/1 -> Product/2
  Product/1 -> Multiply1/1
  Multiply1/1 -> Sum/1
  Multiply/1 -> Sum/2
  Constant/1 -> Sum/3
  Sum/1 -> Simple Actuator leading-edge flap (1st-order dynamics)/1
  Simple Actuator leading-edge flap (1st-order dynamics)/1 -> dlef/1

== system F16_dynamic_model_2019a/MODEL/gravity ==
  In1 : Inport
  Product : Product
  gravity : Constant  Value=9.81
  gravity_body_axis : Subsystem
  mass : Constant  Value=9951
  Out1 : Outport
  Out2 : Outport  Port=2
  wires:
  gravity/1 -> gravity_body_axis/1(gravity)
  gravity_body_axis/1(gravity_body) -> Product/2
  mass/1 -> Out2/1, Product/1
  Product/1 -> Out1/1
  In1/1 -> gravity_body_axis/2("phi theta psi ")

== system F16_dynamic_model_2019a/Subsystem3/Subsystem2 ==
  In1 : Inport
  Add : Sum
  Constant : Constant
  Multiply2 : Gain  Gain=-1
  Multiply4 : Gain  Gain=1/2
  Out1 : Outport
  wires:
  Constant/1 -> Add/2
  Multiply2/1 -> Add/1
  Add/1 -> Multiply4/1
  In1/1 -> Multiply2/1
  Multiply4/1 -> Out1/1

== system F16_dynamic_model_2019a/controller and servo /Gain Scheduling Pitch Rate Feedback ==
  note: NOT: Hız (98-156m/s arası) arttıkça gain azalıyor.
      | Gerçeğinden daha az görüyorum.
  feedback : Inport
  Product3 : Product
  pitch-rate gain (q N/m) : Lookup_n-D  NumberOfTableDimensions=1  BreakpointsForDimension1=[6000, 15000]  Table=[1, 0.3]  ExtrapMethod=Clip  UseLastTableValue=on  InternalRulePriority=Speed  RndMeth=Simplest
  scheduled q feedback : Outport
  wires:
  [q_dyn] -> pitch-rate gain (q N/m)/1
  pitch-rate gain (q N/m)/1 -> Product3/2
  feedback/1 -> Product3/1
  Product3/1 -> scheduled q feedback/1  "feedback"

== system F16_dynamic_model_2019a/controller and servo /Subsystem2 ==
  Pitch rate feedback : Inport
  aoa : Inport  Port=2
  Constant6 : Constant
  Gain : Gain  Gain=0.1
  Product : Product
  Switch5 : Switch  Criteria=u2 > Threshold  Threshold=10  SaturateOnIntegerOverflow=off  InputSameDT=off
  Out1 : Outport
  wires:
  Constant6/1 -> Switch5/3
  aoa/1 -> Switch5/2, Gain/1
  Switch5/1 -> Product/2
  Gain/1 -> Switch5/1
  Pitch rate feedback/1 -> Product/1
  Product/1 -> Out1/1

== system F16_dynamic_model_2019a/controller and servo /scheduled gain ==
  In1 : Inport
  In2 : Inport  Port=2
  1-D Lookup Table : Lookup_n-D  NumberOfTableDimensions=1  BreakpointsForDimension1=[30, 50]  Table=[0 ,1]  ExtrapMethod=Clip  UseLastTableValue=on  InternalRulePriority=Speed  RndMeth=Simplest
  Abs : Abs  SaturateOnIntegerOverflow=off
  Product : Product
  Out1 : Outport
  wires:
  1-D Lookup Table/1 -> Product/2
  Abs/1 -> 1-D Lookup Table/1
  In2/1 -> Abs/1
  Product/1 -> Out1/1
  In1/1 -> Product/1

== system F16_dynamic_model_2019a/controller and servo /servo  ==
  In1 : Inport
  In2 : Inport  Port=2
  In3 : Inport  Port=3
  In4 : Inport  Port=4
  Simple Actuator aileron (1st-order dynamics)1 : aerosimlib/Actuators/Simple Actuator (1st-order dynamics)  MaxRate=80  CountRange=[-21.5 21.5]  ActRange=[-21.5 21.5]  Lag=0.0495
  Simple Actuator elevator (1st-order dynamics) : aerosimlib/Actuators/Simple Actuator (1st-order dynamics)  MaxRate=60  CountRange=[-25 25]  ActRange=[-25 25]  Lag=0.0495
  Simple Actuator rudder (1st-order dynamics)2 : aerosimlib/Actuators/Simple Actuator (1st-order dynamics)  MaxRate=120  CountRange=[-30 30]  ActRange=[-30 30]  Lag=0.0495
  Simple Actuator speed brake (1st-order dynamics)1 : aerosimlib/Actuators/Simple Actuator (1st-order dynamics)  MaxRate=40  CountRange=[0 1]  ActRange=[0 60]  Lag=0.3
  Out1 : Outport
  Out2 : Outport  Port=2
  Out3 : Outport  Port=3
  Output : Outport  Port=4
  wires:
  Simple Actuator rudder (1st-order dynamics)2/1 -> Out3/1
  In2/1 -> Simple Actuator elevator (1st-order dynamics)/1
  In3/1 -> Simple Actuator rudder (1st-order dynamics)2/1
  Simple Actuator elevator (1st-order dynamics)/1 -> Out2/1
  Simple Actuator aileron (1st-order dynamics)1/1 -> Out1/1
  In1/1 -> Simple Actuator aileron (1st-order dynamics)1/1
  In4/1 -> Simple Actuator speed brake (1st-order dynamics)1/1
  Simple Actuator speed brake (1st-order dynamics)1/1 -> Output/1

== system F16_dynamic_model_2019a/MODEL/6-DOF Model Body Euler/Angular_Accel ==
  Moments : Inport
  Inertia : Inport  Port=2
  p q r : Inport  Port=3
  Cross Product : vrlib/Utilities/Cross Product
      settings: SourceProductName=Simulink
  Invert 3x3 Matrix : aerolibutil/Invert  3x3 Matrix
  Matrix Multiply : Product  Multiplication=Matrix(*)
  Matrix Multiply1 : Product  Multiplication=Matrix(*)
  Sum : Sum  Inputs=+-
  "pdot qdot rdot " : Outport
  wires:
  Moments/1 -> Sum/1
  p q r/1 -> Matrix Multiply/2, Cross Product/1
  Inertia/1 -> Matrix Multiply/1, Invert 3x3 Matrix/1
  Matrix Multiply/1 -> Cross Product/2
  Cross Product/1 -> Sum/2
  Invert 3x3 Matrix/1 -> Matrix Multiply1/1
  Sum/1 -> Matrix Multiply1/2
  Matrix Multiply1/1 -> "pdot qdot rdot "/1

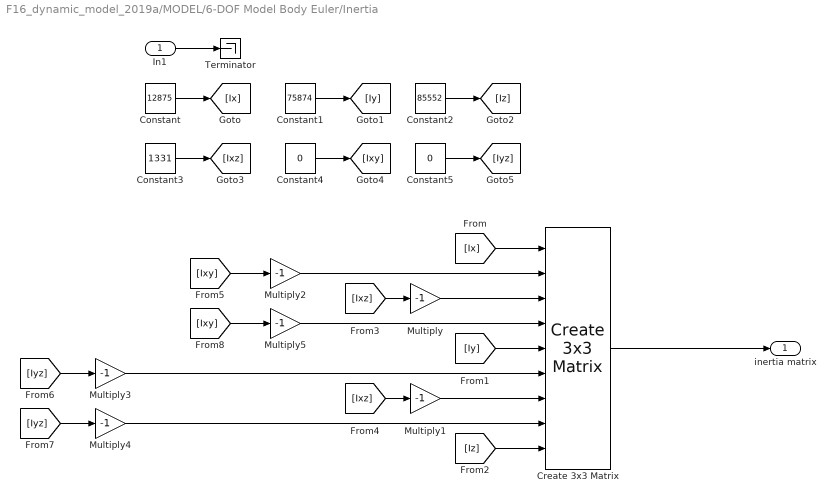
== system F16_dynamic_model_2019a/MODEL/6-DOF Model Body Euler/Inertia ==
  In1 : Inport
  Constant : Constant  Value=12875
  Constant1 : Constant  Value=75874
  Constant2 : Constant  Value=85552
  Constant3 : Constant  Value=1331
  Constant4 : Constant  Value=0
  Constant5 : Constant  Value=0
  Create 3x3 Matrix : sharedutil/Create 3x3 Matrix  aMode=aMode
  Multiply{,1..5} (6 alike) : Gain  Gain=-1
  Terminator : Terminator
  inertia matrix : Outport
  wires:
  In1/1 -> Terminator/1
  Constant/1 -> [Ix]
  Constant1/1 -> [Iy]
  Constant2/1 -> [Iz]
  Constant3/1 -> [Ixz]
  Create 3x3 Matrix/1 -> inertia matrix/1
  [Ix] -> Create 3x3 Matrix/1
  Constant4/1 -> [Ixy]
  Constant5/1 -> [Iyz]
  [Iy] -> Create 3x3 Matrix/5
  [Iz] -> Create 3x3 Matrix/9
  [Ixz] -> Multiply/1
  Multiply/1 -> Create 3x3 Matrix/3
  [Ixz] -> Multiply1/1
  Multiply1/1 -> Create 3x3 Matrix/7
  Multiply2/1 -> Create 3x3 Matrix/2
  [Ixy] -> Multiply2/1
  [Iyz] -> Multiply3/1
  Multiply3/1 -> Create 3x3 Matrix/6
  Multiply4/1 -> Create 3x3 Matrix/8
  [Iyz] -> Multiply4/1
  [Ixy] -> Multiply5/1
  Multiply5/1 -> Create 3x3 Matrix/4

== system F16_dynamic_model_2019a/MODEL/6-DOF Model Body Euler/Subsystem ==
  p q r : Inport
  Quaternions to Direction Cosine Matrix : sharedtransform/Quaternions to  Direction Cosine Matrix  aMode=aMode
      settings: SourceProductName=Aerospace Blockset
  Quaternions to Rotation Angles : sharedtransform/Quaternions to Rotation Angles  rotationOrder=ZYX  aMode=aMode
  Rotation Angles to Quaternions : sharedtransform/Rotation Angles to Quaternions  rotationOrder=ZYX  aMode=aMode
      settings: SourceProductName=Aerospace Blockset
  Selector : Selector  InputPortWidth=3  IndexOptions=Index vector (dialog)  Indices=[3 2 1]  OutputSizes=1
  Selector1 : Selector  InputPortWidth=3  IndexOptions=Index vector (dialog)  Indices=[3 2 1]  OutputSizes=1
  Subsystem : Subsystem
  initial euler : Constant  Value=[0 0 0]
  q0 q1 q2 q3 : Integrator  InitialConditionSource=external  InitialCondition=[e0_0 e1_0 e2_0 e3_0]
  DCM1 : Outport  VectorParamsAs1DForOutWhenUnconnected=off
  Euler : Outport  Port=2  VectorParamsAs1DForOutWhenUnconnected=off
  wires:
  Rotation Angles to Quaternions/1 -> q0 q1 q2 q3/2
  Subsystem/1(qdot) -> q0 q1 q2 q3/1
  initial euler/1 -> Selector1/1
  q0 q1 q2 q3/1 -> Quaternions to Direction Cosine Matrix/1, Quaternions to Rotation Angles/1, Subsystem/2(q0 q1 q2 q3)
  p q r/1 -> Subsystem/1(p q r)
  Quaternions to Direction Cosine Matrix/1 -> DCM1/1
  Selector/1 -> Euler/1
  Quaternions to Rotation Angles/1 -> Selector/1
  Selector1/1 -> Rotation Angles to Quaternions/1

== system F16_dynamic_model_2019a/MODEL/6-DOF Model Body Euler/body_axis_coriolis_accel ==
  u v w : Inport
  p q r : Inport  Port=2
  Add : Sum  Inputs=+-
  Add1 : Sum  Inputs=+-
  Add2 : Sum  Inputs=+-
  Cross Product : vrlib/Utilities/Cross Product
      settings: SourceProductName=Simulink
  Demux : Demux  Outputs=3
  Demux1 : Demux  Outputs=3
  Multiply : Gain  Gain=-1
  Mux : Mux  Inputs=3
  Product{,1..5} (6 alike) : Product
  Terminator : Terminator
  Accel_coriolis_body : Outport
  wires:
  Demux1/3 -> Product/1, Product3/1
  Demux/2 -> Product/2, Product5/2
  Demux1/2 -> Product1/1, Product4/1
  Demux/3 -> Product2/2, Product1/2
  Add/1 -> Mux/1
  Product/1 -> Add/1
  Product1/1 -> Add/2
  Demux1/1 -> Product2/1, Product5/1
  Demux/1 -> Product4/2, Product3/2
  Product2/1 -> Add1/1
  Product3/1 -> Add1/2
  Add1/1 -> Mux/2
  Product5/1 -> Add2/2
  Product4/1 -> Add2/1
  Add2/1 -> Mux/3
  p q r/1 -> Cross Product/1, Demux1/1
  u v w/1 -> Cross Product/2, Demux/1
  Cross Product/1 -> Multiply/1
  Mux/1 -> Accel_coriolis_body/1
  Multiply/1 -> Terminator/1

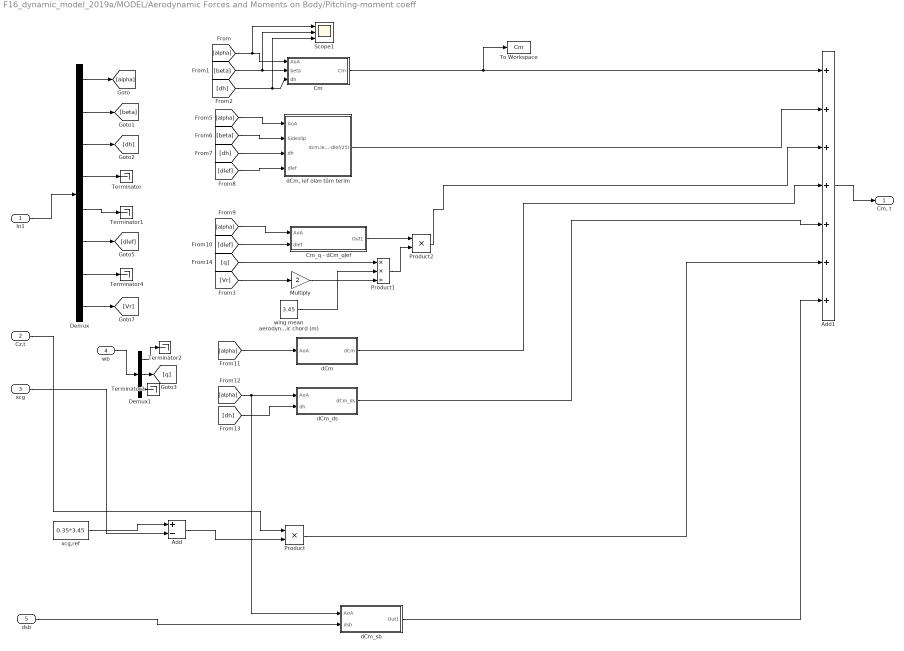
== system F16_dynamic_model_2019a/MODEL/Aerodynamic Forces and Moments on Body/Pitching-moment coeff ==
  In1 : Inport
  Cz,t : Inport  Port=2
  xcg : Inport  Port=3
  wb : Inport  Port=4
  dsb : Inport  Port=5
  Add : Sum  Inputs=+-
  Add1 : Sum  Inputs=+++++++
  Cm : Subsystem
  Cm_q - dCm_qlef : Subsystem
  Demux : Demux  Outputs=8
  Demux1 : Demux  Outputs=3
  Multiply : Gain  Gain=2
  Product : Product
  Product1 : Product  Inputs=**/
  Product2 : Product
  Scope1 : Scope  NumInputPorts=3
  Terminator{,1..4} (5 alike) : Terminator
  To Workspace : ToWorkspace  VariableName=Cm  SampleTime=-1
  dCm : Subsystem
  "dCm, lef olan tüm terim" : Subsystem
  dCm_ds : Subsystem
  dCm_sb : Subsystem
  wing mean aerodynamic chord (m) : Constant  Value=3.45
  xcg,ref : Constant  Value=0.35*3.45
  "Cm, t" : Outport
  wires:
  In1/1 -> Demux/1
  Demux/1 -> [alpha]
  Demux/2 -> [beta]
  Demux/3 -> [dh]
  Demux/4 -> Terminator/1
  Demux/5 -> Terminator1/1
  Cz,t/1 -> Product/1
  xcg,ref/1 -> Add/1
  xcg/1 -> Add/2
  Add/1 -> Product/2
  Cm/1(Cm) -> To Workspace/1, Add1/1
  Add1/1 -> "Cm, t"/1
  [alpha] -> "dCm, lef olan tüm terim"/1(AoA)
  [beta] -> "dCm, lef olan tüm terim"/2("Sideslip ")
  [dh] -> "dCm, lef olan tüm terim"/3(dh)
  Demux/6 -> [dlef]
  [dlef] -> "dCm, lef olan tüm terim"/4(dlef)
  "dCm, lef olan tüm terim"/1(dcm,lef * (1-dlef/25)) -> Add1/2
  [dlef] -> Cm_q - dCm_qlef/2(dlef)
  Cm_q - dCm_qlef/1(Out1) -> Product2/1
  [alpha] -> Cm_q - dCm_qlef/1(AoA)
  wing mean aerodynamic chord (m)/1 -> Product1/2
  Product1/1 -> Product2/2
  Multiply/1 -> Product1/3
  [q] -> Product1/1
  [Vr] -> Multiply/1
  Product2/1 -> Add1/3
  Demux/7 -> Terminator4/1
  Demux/8 -> [Vr]
  [alpha] -> dCm/1(AoA)
  dCm/1(dCm) -> Add1/4
  [alpha] -> dCm_sb/1(AoA), dCm_ds/1(AoA)
  [dh] -> dCm_ds/2(dh)
  dCm_ds/1(dCm_ds) -> Add1/5
  [alpha] -> Scope1/1, Cm/1(AoA)
  [beta] -> Scope1/2, Cm/2(beta)
  [dh] -> Scope1/3, Cm/3(dh)
  Demux1/2 -> [q]
  Demux1/1 -> Terminator2/1
  wb/1 -> Demux1/1
  Demux1/3 -> Terminator3/1
  dsb/1 -> dCm_sb/2(dsb)
  dCm_sb/1(Out1) -> Add1/7
  Product/1 -> Add1/6

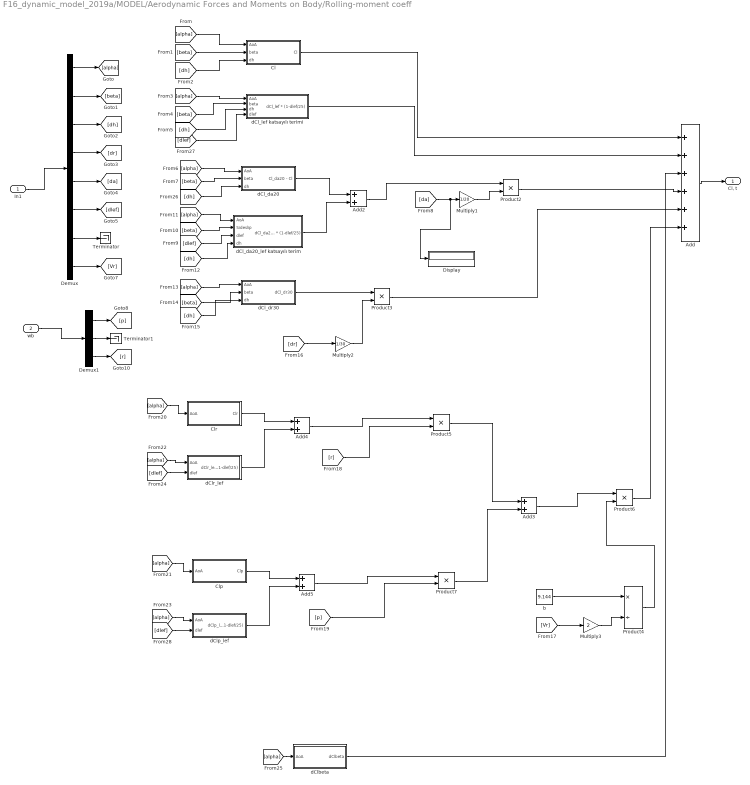
== system F16_dynamic_model_2019a/MODEL/Aerodynamic Forces and Moments on Body/Rolling-moment coeff ==
  In1 : Inport
  wb : Inport  Port=2
  Add : Sum  Inputs=++++++
  Add{2..5} (4 alike) : Sum
  Cl : Subsystem
  Clp : Subsystem
  Clr : Subsystem
  Demux : Demux  Outputs=8
  Demux1 : Demux  Outputs=3
  Display : Display
  Multiply1 : Gain  Gain=1/20
  Multiply2 : Gain  Gain=1/30
  Multiply3 : Gain  Gain=2
  Product{2..3,5..7} (5 alike) : Product
  Product4 : Product  Inputs=*/
  Terminator : Terminator
  Terminator1 : Terminator
  b : Constant  Value=9.144
  dCl_da20 : Subsystem
  dCl_da20_lef katsayılı terim : Subsystem
  dCl_dr30 : Subsystem
  dCl_lef katsayılı terimi : Subsystem
  dClbeta : Subsystem
  dClp_lef : Subsystem
  dClr_lef : Subsystem
  "Cl, t" : Outport
  wires:
  Product2/1 -> Add/4
  [beta] -> Cl/2("beta ")
  Multiply2/1 -> Product3/2
  dCl_dr30/1(dCl_dr30) -> Product3/1
  Add/1 -> "Cl, t"/1
  [dlef] -> dCl_da20_lef katsayılı terim/3(dlef)
  In1/1 -> Demux/1
  Demux/5 -> [da]
  Demux/6 -> [dlef]
  Demux/8 -> [Vr]
  Demux/2 -> [beta]
  Demux/1 -> [alpha]
  wb/1 -> Demux1/1
  Demux/3 -> [dh]
  Demux1/2 -> Terminator1/1
  [alpha] -> dCl_da20_lef katsayılı terim/1(AoA)
  dCl_da20/1(Cl_da20 - Cl) -> Add2/1
  [dr] -> Multiply2/1
  [dlef] -> dClr_lef/2(dlef)
  Product6/1 -> Add/6
  [alpha] -> dClbeta/1(AoA)
  Add4/1 -> Product5/1
  [alpha] -> dClr_lef/1(AoA)
  [dh] -> Cl/3(dh)
  [alpha] -> Clr/1(AoA)
  dCl_da20_lef katsayılı terim/1(dCl_da20lef * (1-dlef/25)) -> Add2/2
  Product5/1 -> Add3/1
  [alpha] -> dClp_lef/1(AoA)
  [alpha] -> dCl_da20/1(AoA)
  Clp/1("Clp ") -> Add5/1
  Add5/1 -> Product7/1
  [r] -> Product5/2
  dClr_lef/1(dClr_lef * (1-dlef/25)) -> Add4/2
  [beta] -> dCl_da20_lef katsayılı terim/2("Sideslip ")
  dClp_lef/1(dClp_lef * (1-dlef/25)) -> Add5/2
  Clr/1(Clr) -> Add4/1
  Product4/1 -> Product6/2
  Multiply3/1 -> Product4/2
  Multiply1/1 -> Product2/2
  b/1 -> Product4/1
  Cl/1(Cl) -> Add/1
  Product7/1 -> Add3/2
  [da] -> Display/1, Multiply1/1
  [dh] -> dCl_dr30/3(dh)
  Product3/1 -> Add/5
  [alpha] -> dCl_lef katsayılı terimi/1(AoA)
  [alpha] -> Clp/1(AoA)
  Add2/1 -> Product2/1
  [beta] -> dCl_lef katsayılı terimi/2(beta)
  [p] -> Product7/2
  [dh] -> dCl_lef katsayılı terimi/3(dh)
  Add3/1 -> Product6/1
  [dh] -> dCl_da20_lef katsayılı terim/4(dh)
  [beta] -> dCl_da20/2(beta)
  [alpha] -> dCl_dr30/1(AoA)
  [beta] -> dCl_dr30/2(beta)
  [alpha] -> Cl/1(AoA)
  Demux1/3 -> [r]
  Demux/4 -> [dr]
  dClbeta/1("dClbeta ") -> Add/3
  dCl_lef katsayılı terimi/1(dCl_lef * (1-dlef/25)) -> Add/2
  Demux/7 -> Terminator/1
  Demux1/1 -> [p]
  [Vr] -> Multiply3/1
  [dh] -> dCl_da20/3(dh)
  [dlef] -> dCl_lef katsayılı terimi/4(dlef)
  [dlef] -> dClp_lef/2(dlef)

== system F16_dynamic_model_2019a/MODEL/Aerodynamic Forces and Moments on Body/X-axis force coeff ==
  In1 : Inport
  wb : Inport  Port=2
  dsb : Inport  Port=3
  Add : Sum  Inputs=++++
  CX_q - dCX_qlef : Subsystem
  Demux : Demux  Outputs=8
  Demux1 : Demux  Outputs=3
  Display : Display
  Multiply : Gain  Gain=2
  Product : Product  Inputs=**/
  Product1 : Product
  Subsystem : Subsystem
  Terminator{,1..4} (5 alike) : Terminator
  "dCX, lef olan tüm terim" : Subsystem
  dCX_sb : Subsystem
  wing mean aerodynamic chord (m) : Constant  Value=3.45
  "CX, t" : Outport
  wires:
  In1/1 -> Demux/1
  Add/1 -> Display/1, "CX, t"/1
  Subsystem/1(Cx) -> Add/1
  "dCX, lef olan tüm terim"/1(dcx,lef * (1-dlef/25)) -> Add/2
  Demux/1 -> dCX_sb/1(AoA), CX_q - dCX_qlef/1(AoA), "dCX, lef olan tüm terim"/1(AoA), Subsystem/1(AoA)
  Demux/2 -> Subsystem/2(Sideslip), "dCX, lef olan tüm terim"/2("Sideslip ")
  Demux/3 -> "dCX, lef olan tüm terim"/3(dh), Subsystem/3(dh)
  Demux/6 -> CX_q - dCX_qlef/2(dlef), "dCX, lef olan tüm terim"/4(dlef)
  CX_q - dCX_qlef/1(Out1) -> Product1/1
  Demux/4 -> Terminator/1
  Demux/5 -> Terminator1/1
  Demux/8 -> Multiply/1
  wing mean aerodynamic chord (m)/1 -> Product/2
  Multiply/1 -> Product/3
  Product/1 -> Product1/2
  Product1/1 -> Add/3
  wb/1 -> Demux1/1
  Demux1/2 -> [q]
  Demux1/1 -> Terminator2/1
  Demux1/3 -> Terminator3/1
  [q] -> Product/1
  Demux/7 -> Terminator4/1
  dsb/1 -> dCX_sb/2(dsb)
  dCX_sb/1(Out1) -> Add/4
